simulink model "simulink_modelo_motor_cc"  (R2017a)
settings: Solver=VariableStepAuto  StartTime=0.0  StopTime=2  RelTol=1e-3
undefined symbols (not defined in the file): b, J, Ke, Kt, La, Ra
settings Model: Creator=bits  LastModifiedBy=bits

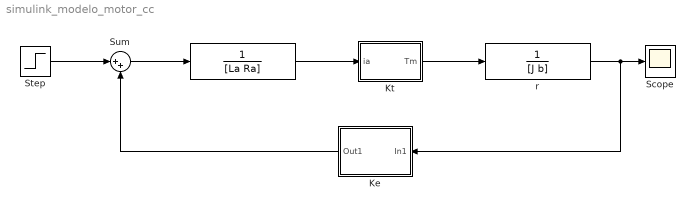
== system simulink_modelo_motor_cc ==
  " " : TransferFcn  Denominator=[La Ra]
  Ke : Subsystem
  Kt : Subsystem
  Scope : Scope
  Step : Step  SampleTime=0
  Sum : Sum  Inputs=|++
  r : TransferFcn  Denominator=[J b]
  wires:
  r/1 -> Scope/1, Ke/1(In1)
  Sum/1 -> " "/1
  " "/1 -> Kt/1(ia)
  Kt/1(Tm) -> r/1
  Ke/1(Out1) -> Sum/2
  Step/1 -> Sum/1

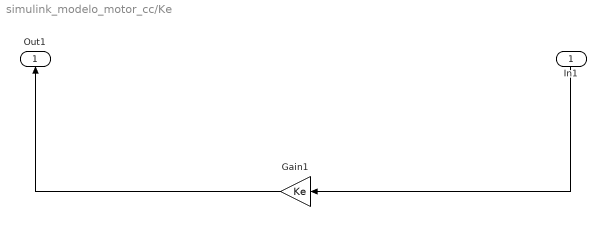
== system simulink_modelo_motor_cc/Ke ==
  In1 : Inport
  Gain1 : Gain  Gain=Ke
  Out1 : Outport
  wires:
  Gain1/1 -> Out1/1
  In1/1 -> Gain1/1

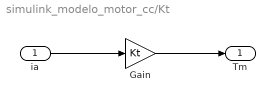
== system simulink_modelo_motor_cc/Kt ==
  ia : Inport
  Gain : Gain  Gain=Kt
  Tm : Outport
  wires:
  Gain/1 -> Tm/1
  ia/1 -> Gain/1
